simulink model "Gaseigenschaften"  (R2024a)
settings: Solver=VariableStepAuto  StartTime=0.0  StopTime=400  RelTol=1e-3
libraries: Bibliothek_FHDO_V1 x11, simulink x3
settings Model: Creator=goessling  LastModifiedBy=goessling

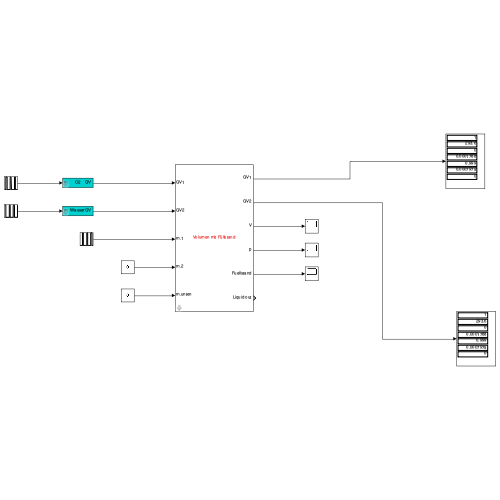
[thumbnail: Simulink's stored preview of the top-level diagram]
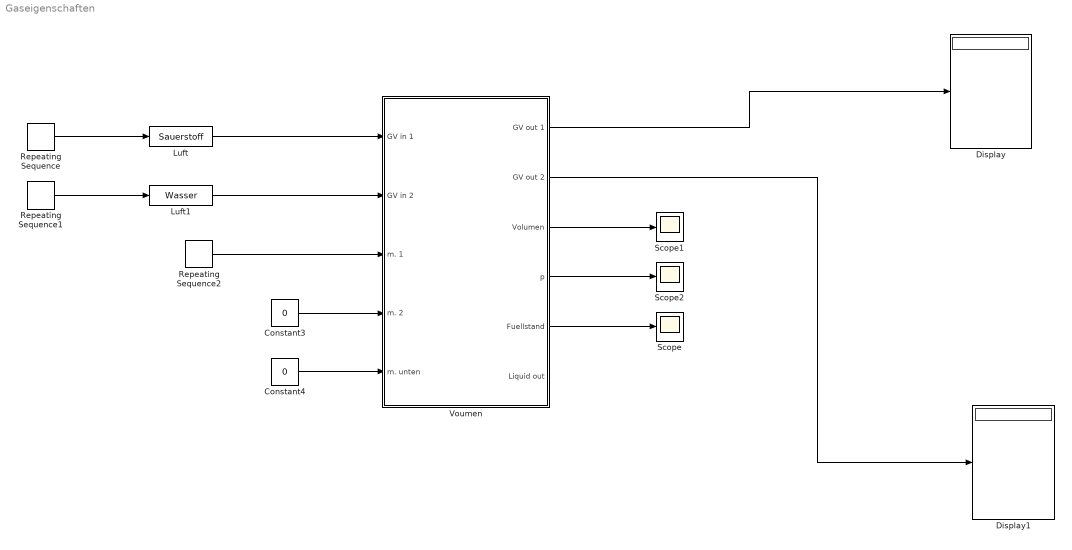
== system Gaseigenschaften ==
  Constant3 : Constant  Value=0
  Constant4 : Constant  Value=0
  Display : Display
  Display1 : Display
  Luft : Bibliothek_FHDO_V1/Sauerstoff  p=1  T=25
  Luft1 : Bibliothek_FHDO_V1/Wasser  p=1  T=25
  Repeating Sequence : simulink/Sources/Repeating Sequence  rep_seq_t=[0 100 100.1 200 200.1 300 300.1 400]  rep_seq_y=[0 0 0.2 0.2 0 0 0 0]
  Repeating Sequence1 : simulink/Sources/Repeating Sequence  rep_seq_t=[0 100 100.1 200 200.1 300 300.1 400]  rep_seq_y=[250 250 0 0 0 0 0 0]
  Repeating Sequence2 : simulink/Sources/Repeating Sequence  rep_seq_t=[0 100 100.1 200 200.1 300 300.1 400]  rep_seq_y=[0 0 0 0 250 250 0 0]
  Scope : Scope
  Scope1 : Scope
  Scope2 : Scope
  Voumen : Subsystem  mask{V=0.1, p_start=1, T_start=25, x_start=[0.1 0.9 0 0]}
      mask prompts: V "Volumen [m^3]"; p_start "p [bar]"; T_start "T [°C]"; x_start "x"
      mask Display:
      | color('red')
      | disp(['Volumen mit Füllstand'])
      | 
      | color('black')
      | port_label('input', 1, 'GV1')
      | port_label('input', 2, 'GV2')
      | port_label('input', 3, 'm.1')
      | port_label('input', 4, 'm.2')
      | port_label('input', 5, 'm.unten')
      | 
      | port_label('output', 1, 'GV1')
      | port_label('output', 2, 'GV2')
      | port_label('output', 3, 'V')
      | port_label('output', 4, 'p')
      | port_label('output', 5, 'Fuellstand')
      | port_label('output', 6, 'Liquid out')
  wires:
  Luft/1 -> Voumen/1(GV in 1)
  Repeating Sequence1/1 -> Luft1/1
  Luft1/1 -> Voumen/2(GV in 2)
  Repeating Sequence/1 -> Luft/1
  Repeating Sequence2/1 -> Voumen/3(m. 1)
  Constant3/1 -> Voumen/4(m. 2)
  Constant4/1 -> Voumen/5(m. unten)
  Voumen/5(Fuellstand) -> Scope/1
  Voumen/3(Volumen) -> Scope1/1
  Voumen/4(p) -> Scope2/1
  Voumen/1(GV out 1) -> Display/1
  Voumen/2(GV out 2) -> Display1/1

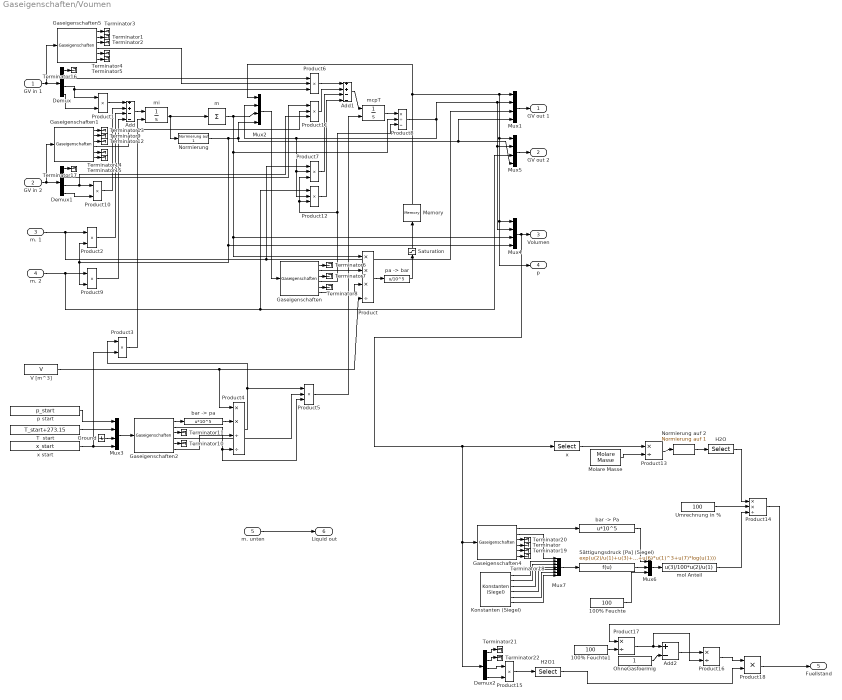
== system Gaseigenschaften/Voumen ==
  GV in 1 : Inport
  GV in 2 : Inport  Port=2
  m. 1 : Inport  Port=3
  m. 2 : Inport  Port=4
  m. unten : Inport  Port=5
  100% Feuchte : Constant  Value=100
  100% Feuchte1 : Constant  Value=100
  Add : Sum  Inputs=++--
  Add1 : Sum  Inputs=++--  SampleTime=.01
  Add2 : Sum  Inputs=+-
  Demux : Demux  Outputs=[1 1 1 4]
  Demux1 : Demux  Outputs=[1 1 1 4]
  Demux2 : Demux  Outputs=[1 1 1 4]
  Gaseigenschaften{,1..2,4..5} (5 alike) : Bibliothek_FHDO_V1/Gaseigenschaften  SystemSampleTime=-1  VariantActivationTime=update diagram  AllowFlexibleInterface=on  Latency=0  AutoFrameSizeCalculation=off
  Ground : Ground
  H2O : Selector  InputPortWidth=4  IndexOptions=Index vector (dialog)  Indices=2  OutputSizes=1
  H2O1 : Selector  InputPortWidth=4  IndexOptions=Index vector (dialog)  Indices=2  OutputSizes=1
  Konstanten (Siegel) : Bibliothek_FHDO_V1/Befeuchter//Abscheider/Konstanten (Siegel)  SystemSampleTime=-1  VariantActivationTime=update diagram  AllowFlexibleInterface=on  Latency=0  AutoFrameSizeCalculation=off
  Memory : Memory  InitialCondition=p_start
  Molare Masse : Bibliothek_FHDO_V1/Molare Masse  SystemSampleTime=-1  VariantActivationTime=update diagram  AllowFlexibleInterface=on  Latency=0  AutoFrameSizeCalculation=off
  Mux{1..5} (5 alike) : Mux
  Mux6 : Mux  Inputs=3
  Mux7 : Mux  Inputs=7
  Normierung : Bibliothek_FHDO_V1/Sauerstoff/Normierung auf 1  SystemSampleTime=-1  VariantActivationTime=update diagram  AllowFlexibleInterface=on  Latency=0  AutoFrameSizeCalculation=off
  Normierung auf 2 : Bibliothek_FHDO_V1/Sauerstoff/Normierung auf 1  SystemSampleTime=-1  VariantActivationTime=update diagram  AllowFlexibleInterface=on  Latency=0  AutoFrameSizeCalculation=off
  OhneGasfoermig : Constant
  Product : Product  Inputs=***/  RndMeth=Zero
  Product{1..3,9..10,15} (6 alike) : Product  RndMeth=Zero
  Product{5..7,11..12} (5 alike) : Product  Inputs=3  RndMeth=Zero
  Product13 : Product  Inputs=*/  RndMeth=Zero
  Product14 : Product  Inputs=**/  RndMeth=Zero
  Product16 : Product  Inputs=*/
  Product17 : Product  Inputs=*/
  Product18 : Product
  Product4 : Product  Inputs=**//  RndMeth=Zero
  Product8 : Product  Inputs=*//  RndMeth=Zero
  Saturation : Saturate  UpperLimit=inf  LowerLimit=1
  Sättigungsdruck [Pa] (Siegel) : Fcn  Expr=exp(u(2)/u(1)+u(3)+u(4)*u(1)+u(5)*u(1)^2+u(6)*u(1)^3+u(7)*log(u(1)))
  T  start : Constant  Value=T_start+273.15
  Terminator{,1..22} (23 alike) : Terminator
  Umrechnung in % : Constant  Value=100
  V [m^3] : Constant  Value=V
  "bar -> Pa" : Fcn  Expr=u*10^5
  "bar -> pa" : Fcn  Expr=u*10^5
  m : Sum  Inputs=+
  mcpT : Integrator  InitialConditionSource=external  InitialCondition=[0 0 0 0 0 0 .21 .79]*1293
  mi : Integrator  InitialConditionSource=external  InitialCondition=[0 0 0 0 0 0 .21 .79]*1293
  mol Anteil : Fcn  Expr=u(3)/100*u(2)/u(1)
  p start : Constant  Value=p_start
  "pa -> bar" : Fcn  Expr=u/10^5
  x : Selector  InputPortWidth=7  IndexOptions=Index vector (dialog)  Indices=[4 5 6 7]  OutputSizes=1
  x start : Constant  Value=x_start
  GV out 1 : Outport
  GV out 2 : Outport  Port=2
  Volumen : Outport  Port=3
  p : Outport  Port=4
  Fuellstand : Outport  Port=5
  Liquid out : Outport  Port=6
  wires:
  GV in 1/1 -> Gaseigenschaften5/1, Demux/1
  Demux/3 -> Product1/1, Product6/3
  Demux/2 -> Product6/1
  Demux/4 -> Product1/2
  Gaseigenschaften/1 -> Terminator6/1
  Gaseigenschaften/4 -> Product8/3, Product7/3, Product12/3
  Product1/1 -> Add/1
  m. 1/1 -> Product2/1, Product7/1, Mux1/3
  mi/1 -> Normierung/1, m/1
  Normierung/1 -> Mux2/4, Mux1/4, Mux5/4, Mux4/4, Product2/2, Product9/2
  Product2/1 -> Add/3
  Add/1 -> mi/1
  m/1 -> Mux2/3, Product8/2, Product/1, Mux4/3
  Mux2/1 -> Gaseigenschaften/1
  Gaseigenschaften5/1 -> Terminator3/1
  Gaseigenschaften5/4 -> Product6/2
  Gaseigenschaften/6 -> Product/3
  Gaseigenschaften/2 -> Product/2
  V [m^3]/1 -> Product4/1, Product/4
  Product/1 -> "pa -> bar"/1
  Mux1/1 -> GV out 1/1
  Gaseigenschaften5/2 -> Terminator1/1
  Gaseigenschaften5/3 -> Terminator2/1
  Gaseigenschaften5/5 -> Terminator4/1
  Gaseigenschaften5/6 -> Terminator5/1
  Gaseigenschaften/3 -> Terminator7/1
  Gaseigenschaften/5 -> Terminator8/1
  "pa -> bar"/1 -> Saturation/1
  x start/1 -> Mux3/4, Product3/2
  Ground/1 -> Mux3/3
  p start/1 -> Mux3/1
  T  start/1 -> Mux3/2
  Mux3/1 -> Gaseigenschaften2/1
  Gaseigenschaften2/1 -> "bar -> pa"/1
  "bar -> pa"/1 -> Product4/2
  Gaseigenschaften2/6 -> Product4/3
  Gaseigenschaften2/2 -> Product4/4, Product5/3
  Gaseigenschaften2/3 -> Terminator11/1
  Gaseigenschaften2/4 -> Product5/2
  Gaseigenschaften2/5 -> Terminator10/1
  Product4/1 -> Product5/1, Product3/1
  Product3/1 -> mi/2
  Product5/1 -> mcpT/2
  Product6/1 -> Add1/1
  Add1/1 -> mcpT/1
  mcpT/1 -> Product8/1
  Product8/1 -> Mux2/2, Product7/2, Product12/2, Mux1/2, Mux4/2, Mux5/2
  Product7/1 -> Add1/3
  m. 2/1 -> Product9/1, Mux5/3, Product12/1
  Product9/1 -> Add/4
  Mux5/1 -> GV out 2/1
  GV in 2/1 -> Gaseigenschaften1/1, Demux1/1
  Gaseigenschaften1/1 -> Terminator13/1
  Gaseigenschaften1/2 -> Terminator9/1
  Gaseigenschaften1/3 -> Terminator12/1
  Gaseigenschaften1/5 -> Terminator14/1
  Gaseigenschaften1/6 -> Terminator15/1
  Demux/1 -> Terminator16/1
  Demux1/1 -> Terminator17/1
  Demux1/3 -> Product10/1, Product11/3
  Demux1/4 -> Product10/2
  Product10/1 -> Add/2
  Product11/1 -> Add1/2
  Product12/1 -> Add1/4
  Gaseigenschaften1/4 -> Product11/2
  Demux1/2 -> Product11/1
  Memory/1 -> Mux1/1, Mux5/1, Mux4/1, p/1, Mux2/1
  Saturation/1 -> Memory/1
  m. unten/1 -> Liquid out/1
  Gaseigenschaften4/6 -> Terminator18/1
  "bar -> Pa"/1 -> Mux6/1
  mol Anteil/1 -> Product14/3
  x/1 -> Product13/1
  Gaseigenschaften4/3 -> Terminator20/1
  Sättigungsdruck [Pa] (Siegel)/1 -> Mux6/2
  H2O/1 -> Product14/1
  Konstanten (Siegel)/6 -> Mux7/7
  Mux4/1 -> x/1, Demux2/1, Gaseigenschaften4/1, Volumen/1
  Gaseigenschaften4/5 -> Terminator19/1
  Product13/1 -> Normierung auf 2/1
  Mux6/1 -> mol Anteil/1
  Normierung auf 2/1 -> H2O/1
  Umrechnung in %/1 -> Product14/2
  Konstanten (Siegel)/2 -> Mux7/3
  Gaseigenschaften4/2 -> Mux7/1
  Mux7/1 -> Sättigungsdruck [Pa] (Siegel)/1
  Gaseigenschaften4/1 -> "bar -> Pa"/1
  100% Feuchte/1 -> Mux6/3
  Konstanten (Siegel)/5 -> Mux7/6
  Gaseigenschaften4/4 -> Terminator/1
  Konstanten (Siegel)/1 -> Mux7/2
  Konstanten (Siegel)/3 -> Mux7/4
  Konstanten (Siegel)/4 -> Mux7/5
  Molare Masse/1 -> Product13/2
  Demux2/3 -> Product15/1
  Demux2/4 -> Product15/2
  Demux2/1 -> Terminator21/1
  Demux2/2 -> Terminator22/1
  Product15/1 -> H2O1/1
  Product14/1 -> Product17/1
  100% Feuchte1/1 -> Product17/2
  Product17/1 -> Product16/2, Add2/1
  OhneGasfoermig/1 -> Add2/2
  Add2/1 -> Product16/1
  Product16/1 -> Product18/1
  H2O1/1 -> Product18/2
  Product18/1 -> Fuellstand/1
